simulink model "figure11with6states"  (R2021a)
settings: Solver=VariableStepAuto  StartTime=0.0  StopTime=10.0  RelTol=1e-3
settings Model: Creator=ibirl  LastModifiedBy=zht

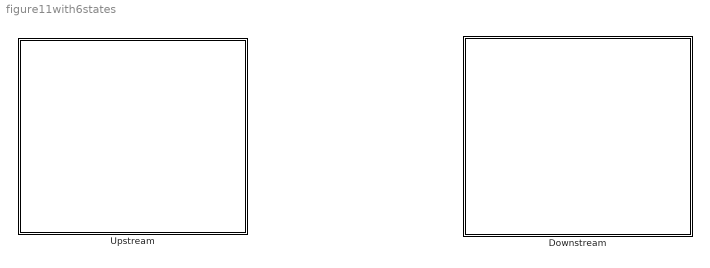
== system figure11with6states ==
  Downstream : Stateflow chart  TreatAsAtomicUnit=on
  Upstream : Stateflow chart  TreatAsAtomicUnit=on

== stateflow chart figure11with6states/Downstream ==
  state E
  state D
  state A
  state B
  state C
  state F
  E -> B [order 3] : (1)[0.9]{0}
  E -> A [order 2] : (1)[0.1*(1-pb)]{-1}
  E -> D [order 1] : (1)[0.1*pb]{-1}
  D -> E [order 1] : (A1)[1-pbd]{0}
  D -> D [order 2] : (1)[pbd]{0}
  C -> D [order 3] : (1)[pb*(1-p)]{-1}
  B -> D [order 4] : (1)[(0.6664)*(1-p)*pb]{-1}
  A -> D [order 3] : (1)[0.1*(1-p)*pb]{-1}
  C -> A [order 2] : (1)[(1-pb)*(1-p)]{-1}
  B -> A [order 3] : (1)[0.6664*(1-p)*(1-pb)]{-1}
  F -> A [order 2] : (1)[r]{0}
  A -> B [order 2] : (0)[(1-p)*0.9]{0}
  B -> C [order 2] : (1)[0.2679*(1-p)]{0}
  A -> A [order 1] : (1)[(1-p)*0.1*(1-pb)]{-1}
  A -> F [order 4] : (1)[p]{0}
  B -> F [order 5] : (1)[p]{0}
  B -> B [order 1] : (1)[0.0657*(1-p)]{0}
  C -> F [order 4] : (1)[p]{0}
  C -> C [order 1] : (1)[0]{0}
  F -> F [order 1] : (1)[1-r]{0}

== stateflow chart figure11with6states/Upstream ==
  state E
  state D
  state A
  state B
  state C
  state F
  E -> B [order 3] : (1)[0.9]{0}
  E -> A [order 2] : (1)[0.1*(1-ps)]{1}
  E -> D [order 1] : (1)[0.1*ps]{1}
  D -> E [order 1] : (A1)[1-psu]{0}
  C -> D [order 3] : (1)[ps*(1-p)]{1}
  D -> D [order 2] : (1)[psu]{0}
  B -> D [order 4] : (1)[(0.6664)*(1-p)*ps]{1}
  C -> A [order 2] : (1)[(1-p)*(1-ps)]{1}
  A -> D [order 3] : (1)[0.1*(1-p)*ps]{1}
  B -> A [order 3] : (1)[0.6664*(1-p)*(1-ps)]{1}
  A -> B [order 2] : (0)[0.9*(1-p)]{0}
  B -> C [order 2] : (1)[0.2679*(1-p)]{0}
  A -> F [order 4] : (1)[p]{0}
  F -> A [order 2] : (1)[r]{0}
  A -> A [order 1] : (1)[0.1*(1-p)*(1-ps)]{1}
  B -> F [order 5] : (1)[p]{0}
  B -> B [order 1] : (1)[0.0657*(1-p)]{0}
  C -> F [order 4] : (1)[p]{0}
  C -> C [order 1] : (1)[0]{0}
  F -> F [order 1] : (1)[1-r]{0}
